simulink model "Para_sacar_imagenes"  (R2018a)
settings: Solver=VariableStepAuto  StartTime=0.0  StopTime=10.0  RelTol=1e-3
libraries: simulink x1
settings Model: Creator=quich  LastModifiedBy=quich

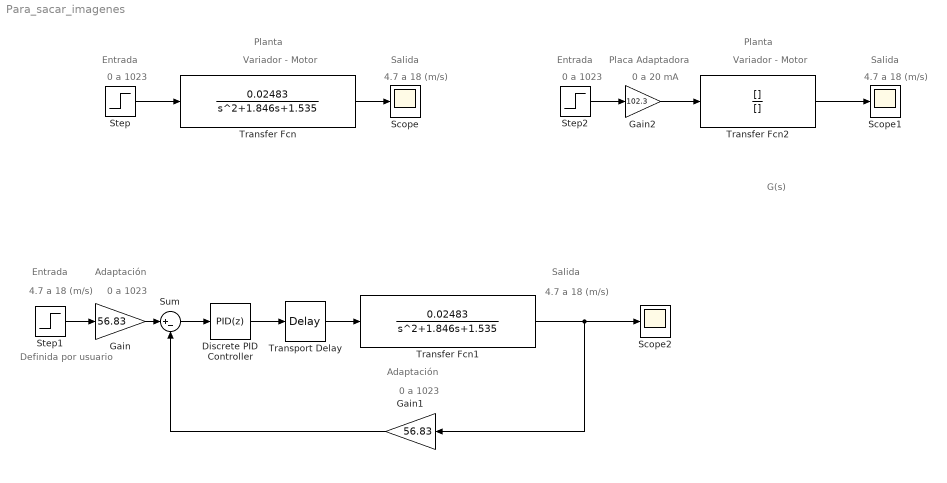
== system Para_sacar_imagenes ==
  note: G(s)
  note: Entrada
  note: 0 a 1023
  note: Salida
  note: 4.7 a 18 (m/s)
  note: Planta
  note: Variador - Motor
  note: Planta
  note: Salida
  note: 4.7 a 18 (m/s)
  note: Variador - Motor
  note: Entrada
  note: 0 a 1023
  note: 0 a 20 mA
  note: Placa Adaptadora
  note: 4.7 a 18 (m/s)
  note: Entrada
  note: Definida por usuario
  note: Adaptación
  note: 0 a 1023
  note: Salida
  note: 4.7 a 18 (m/s)
  note: 0 a 1023
  note: Adaptación
  Discrete PID Controller : simulink/Continuous/PID Controller  Controller=PID  TimeDomain=Discrete-time  SampleTime=-1  IntegratorMethod=Forward Euler  FilterMethod=Forward Euler  Form=Parallel  UseFilter=on  ControllerParametersSource=internal  P=1  I=1  D=0  N=100  InitialConditionSource=internal  InitialConditionForIntegrator=0  InitialConditionForFilter=0  ExternalReset=none  LimitOutput=off  UpperSaturationLimit=inf  LowerSaturationLimit=-inf  LinearizeAsGain=off  AntiWindupMode=none  Kb=1  TrackingMode=off  Kt=1  PParamMin=[]  PParamMax=[]  IParamMin=[]  IParamMax=[]  DParamMin=[]  DParamMax=[]  NParamMin=[]  NParamMax=[]  KbParamMin=[]  KbParamMax=[]  KtParamMin=[]  KtParamMax=[]  POutMin=[]  POutMax=[]  IOutMin=[]  IOutMax=[]  DOutMin=[]  DOutMax=[]  NOutMin=[]  NOutMax=[]  KbOutMin=[]  KbOutMax=[]  KtOutMin=[]  KtOutMax=[]  IntegratorOutMin=[]  IntegratorOutMax=[]  FilterOutMin=[]  FilterOutMax=[]  SumOutMin=[]  SumOutMax=[]  SumI1OutMin=[]  SumI1OutMax=[]  SumI2OutMin=[]  SumI2OutMax=[]  SumI3OutMin=[]  SumI3OutMax=[]  SumDOutMin=[]  SumDOutMax=[]  SaturationOutMin=[]  SaturationOutMax=[]  IntegratorContinuousStateAttributes=''  IntegratorStateMustResolveToSignalObject=off  IntegratorRTWStateStorageClass=Auto  FilterContinuousStateAttributes=''  FilterStateMustResolveToSignalObject=off  FilterRTWStateStorageClass=Auto  DifferentiatorICPrevScaledInput=0  DifferentiatorOutMin=[]  DifferentiatorOutMax=[]  FilterDiffOutCoefMin=[]  FilterDiffOutCoefMax=[]  SumDenOutMin=[]  SumDenOutMax=[]  SumNumOutMin=[]  SumNumOutMax=[]  ReciprocalOutMin=[]  ReciprocalOutMax=[]  DivideOutMin=[]  DivideOutMax=[]  TunerSelectOption=Transfer Function Based (PID Tuner App)
  Gain : Gain  Gain=56.83
  Gain1 : Gain  Gain=56.83
  Gain2 : Gain  Gain=102.3
  Scope : Scope
  Scope1 : Scope
  Scope2 : Scope
  Step : Step  Time=2  After=1023  SampleTime=0
  Step1 : Step  Time=2  After=1023  SampleTime=0
  Step2 : Step  Time=2  After=1023  SampleTime=0
  Sum : Sum  Inputs=|+-
  Transfer Fcn : TransferFcn  Numerator=[0.02483]  Denominator=[1 1.846 1.535]
  Transfer Fcn1 : TransferFcn  Numerator=[0.02483]  Denominator=[1 1.846 1.535]
  Transfer Fcn2 : TransferFcn  Numerator=[]  Denominator=[]  ContinuousStateAttributes='G(s)'
  Transport Delay : TransportDelay  DelayTime=1.2
  wires:
  Transfer Fcn/1 -> Scope/1
  Step1/1 -> Gain/1
  Gain/1 -> Sum/1
  Sum/1 -> Discrete PID Controller/1
  Transfer Fcn1/1 -> Gain1/1, Scope2/1
  Gain1/1 -> Sum/2
  Step/1 -> Transfer Fcn/1
  Transfer Fcn2/1 -> Scope1/1
  Step2/1 -> Gain2/1
  Gain2/1 -> Transfer Fcn2/1
  Discrete PID Controller/1 -> Transport Delay/1
  Transport Delay/1 -> Transfer Fcn1/1
